simulink model "Furuta_Control_all_states_24_12_4am0x2810x29"  (R2023b)
settings: Solver=FixedStepAuto  StartTime=0.0  StopTime=inf  FixedStep=Ts  RelTol=1e-3
PreLoadFcn:
  | %myBusDef
StartFcn:
  | % Full path to the block
  | %blk = 'Furuta_Control/Bus Creator';
  | 
  | % Attach the event listener
  | %h = add_exec_event_listener(blk, ...
  | %         'PostOutputs', @displayBusdata);
values from neighbouring files (symbols this model uses):
  a = exp(-wc*Ts)    [Furuta_Constants.m]
  K2 = place(Ap2,Bp2,[-5 -4 -2+2j -2-2j])    [Furuta_Constants.m]
libraries: arduinolib x3, eeGeneralControl x2, arduinosensorlib x2
settings Model: ExtModeTrigDuration=2  Creator=Marcelo  LastModifiedBy=Omar Elshawaf
settings SolverCC: ZeroCrossControl=DisableAll  AlgebraicLoopSolver=TrustRegion
settings DataIOCC: ReturnWorkspaceOutputs=off
settings OptimizationCC: EnhancedBackFolding=on  PassReuseOutputArgsAs=Individual arguments  ZeroExternalMemoryAtStartup=off  ZeroInternalMemoryAtStartup=off  MaxStackSize=64  OptimizeBlockOrder=speed  DifferentSizesBufferReuse=on  OptimizationCustomize=off  EfficientTunableParamExpr=on
settings DebuggingCC: ParameterOverflowMsg=warning  ParameterTunabilityLossMsg=error  UnconnectedInputMsg=warning  UnconnectedOutputMsg=warning  UnconnectedLineMsg=warning  BusObjectLabelMismatch=error  ArithmeticOperatorsInVariantConditions=warning
settings HardwareCC: ProdBitPerPointer=32  ProdBitPerSizeT=32  ProdBitPerPtrDiffT=32  ProdLargestAtomicInteger=Long  ProdLargestAtomicFloat=Double  ProdWordSize=32  ProdHWDeviceType=ARM Compatible->ARM Cortex
settings ModelReferenceCC: EnableRefExpFcnMdlSchedulingChecks=on  ModelReferenceMinAlgLoopOccurrences=on
settings SFSimCC: SimUseLocalCustomCode=off  MATLABDynamicMemAlloc=off  CustomCodeUndefinedFunction=UseInterfaceOnly
settings RTWCC: Description=Embedded Coder  SystemTargetFile=ert.tlc  HardwareBoard=ESP32-WROOM(Arduino Compatible)  TLCOptions="-aInlineSetEventsForThisBaseRateFcn=TLC_FALSE -aSuppressMultiTaskScheduler=TLC_FALSE  -aRateBasedStepFcn=0"  TemplateMakefile=ert_default_tmf  RTWUseLocalCustomCode=off  Toolchain=ESP32
settings CodeAppCC: ForceParamTrailComments=on  IgnoreCustomStorageClasses=off  OperatorAnnotations=on  SimulinkDataObjDesc=on  SFDataObjDesc=on  InsertBlockDesc=on
settings ERTTargetCC: SupportContinuousTime=on  SupportVariableSizeSignals=on  ExtModeTransport=3  ExtModeStaticAlloc=on  ExtModeAutomaticAllocSize=off  ExtModeStaticAllocSize=65536  ExtModeMexFile=ext_xcp  ExtModeMexArgs=0 12 115200  ExtModeIntrfLevel=Level2 - Open

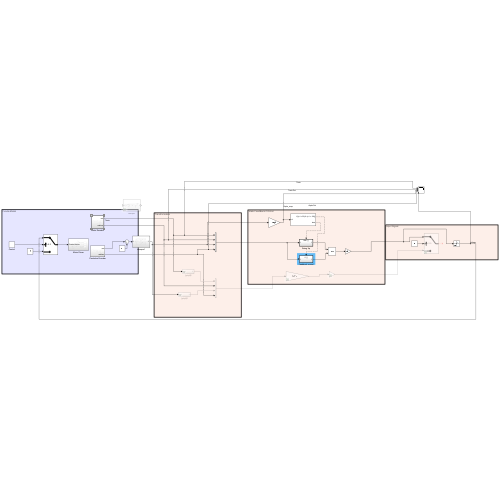
[thumbnail: Simulink's stored preview of the top-level diagram]
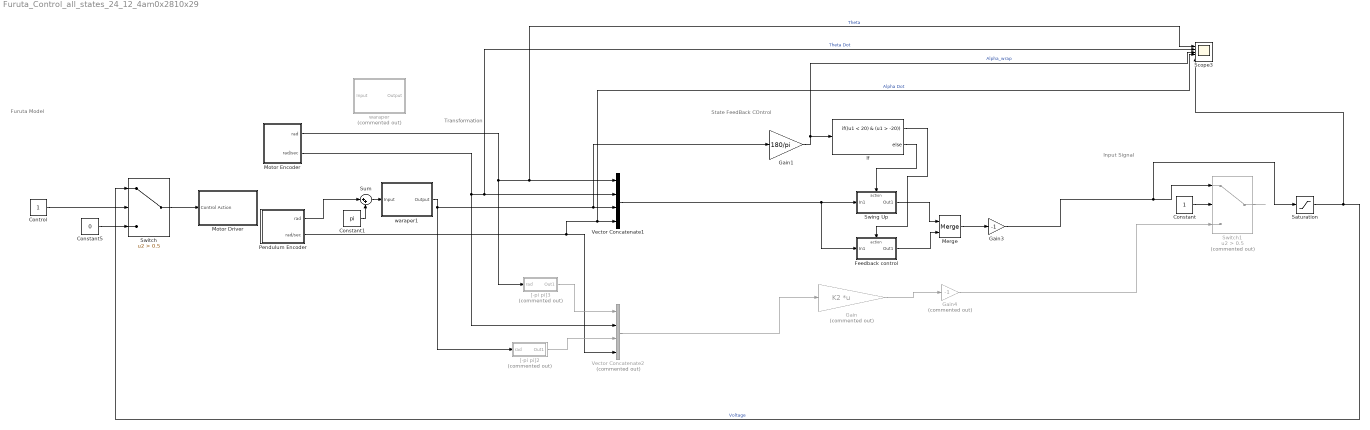
== system Furuta_Control_all_states_24_12_4am0x2810x29 ==
  note: State FeedBack COntrol
  note: Input Signal
  note: Furuta Model
  note: Transformation
  Constant : Constant  SampleTime=-1
  Constant1 : Constant  Value=pi  SampleTime=-1
  Constant5 : Constant  Value=0
  Control : Constant  SampleTime=-1
  Feedback control : Subsystem  TreatAsAtomicUnit=on
  Gain : Gain  Commented=on  Gain=K2  Multiplication=Matrix(K*u)
  Gain1 : Gain  Gain=180/pi
  Gain3 : Gain  Gain=-1
  Gain4 : Gain  Commented=on  Gain=-1
  If : If  IfExpression=(u1 < 20) & (u1 > -20)
  Merge : Merge
  Motor Driver : Subsystem
  Motor Encoder : Subsystem
  Pendulum Encoder : Subsystem
  Saturation : Saturate  UpperLimit=255  LowerLimit=-255
  Scope3 : Scope  NumInputPorts=5
  Sum : Sum  Inputs=|++
  Swing Up : Subsystem  TreatAsAtomicUnit=on
  Switch : Switch  Criteria=u2 > Threshold  Threshold=0.5  SaturateOnIntegerOverflow=off  InputSameDT=off
  Switch1 : Switch  Commented=on  Criteria=u2 > Threshold  Threshold=0.5  SaturateOnIntegerOverflow=off  InputSameDT=off
  Vector Concatenate1 : Concatenate  NumInputs=4  Mode=Multidimensional array
  Vector Concatenate2 : Concatenate  Commented=on  NumInputs=4  Mode=Multidimensional array
  "[-pi pi]2" : Subsystem  Commented=on
  "[-pi pi]3" : Subsystem  Commented=on
  waraper : Subsystem  Commented=on
  waraper1 : Subsystem
  wires:
  Swing Up/1(Out1) -> Merge/1
  Pendulum Encoder/2(rad/sec) -> Vector Concatenate2/4, Scope3/4, Vector Concatenate1/4  "Alpha Dot"
  Feedback control/1(Out1) -> Merge/2
  Control/1 -> Switch/2
  Constant5/1 -> Switch/3
  Sum/1 -> waraper1/1(Input)
  Vector Concatenate1/1 -> Feedback control/1(In1), Swing Up/1(In1)
  Gain1/1 -> Scope3/3, If/1  "Alpha_wrap"
  "[-pi pi]2"/1(Out1) -> Vector Concatenate2/3
  Motor Encoder/2(rad/sec) -> Vector Concatenate2/2, Vector Concatenate1/2, Scope3/2  "Theta Dot"
  Vector Concatenate2/1 -> Gain/1
  Saturation/1 -> Switch/1, Scope3/5  "Voltage"
  Switch1/1 -> ?
  Gain3/1 -> Saturation/1, Switch1/1
  Gain4/1 -> Switch1/3
  Merge/1 -> Gain3/1
  Constant/1 -> Switch1/2
  Switch/1 -> Motor Driver/1(Control Action)
  Gain/1 -> Gain4/1
  "[-pi pi]3"/1(Out1) -> Vector Concatenate2/1
  If/2 -> Swing Up/Action
  If/1 -> Feedback control/Action
  Constant1/1 -> Sum/2
  Pendulum Encoder/1(rad) -> Sum/1
  waraper1/1(Output) -> "[-pi pi]2"/1(rad), Gain1/1, Vector Concatenate1/3
  Motor Encoder/1(rad) -> Vector Concatenate1/1, Scope3/1, "[-pi pi]3"/1(rad)  "Theta"

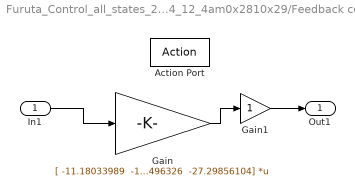
== system Furuta_Control_all_states_24_12_4am0x2810x29/Feedback control ==
  In1 : Inport
  Action Port : ActionPort  ActionPortLabel=if((u1 < 20) & (u1 > -20))
  Gain : Gain  Gain="[ -11.18033989  -17.56383192 -336.55496326  -27.29856104]"  Multiplication=Matrix(K*u)  ParamDataTypeStr=double  OutDataTypeStr=double
  Gain1 : Gain
  Out1 : Outport  VectorParamsAs1DForOutWhenUnconnected=off
  wires:
  In1/1 -> Gain/1
  Gain/1 -> Gain1/1
  Gain1/1 -> Out1/1

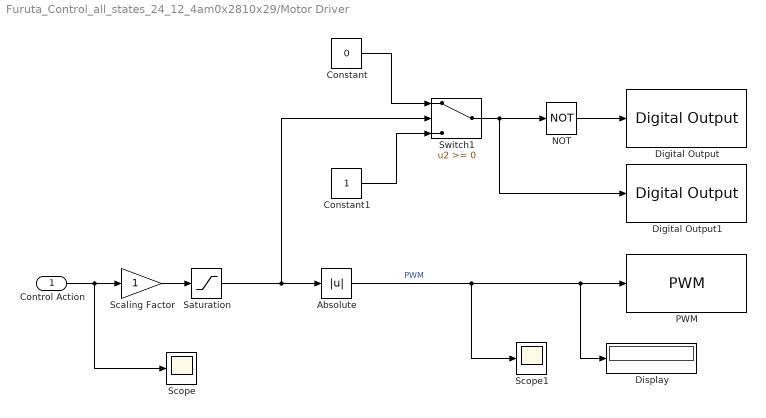
== system Furuta_Control_all_states_24_12_4am0x2810x29/Motor Driver ==
  Control Action : Inport
  Absolute : Abs  SaturateOnIntegerOverflow=off
  Constant : Constant  Value=0
  Constant1 : Constant
  Digital Output : arduinolib/Digital Output  pinNumber=26  Direction=output  blockPlatform=arduino
  Digital Output1 : arduinolib/Digital Output  pinNumber=19  Direction=output  blockPlatform=arduino
  Display : Display
  NOT : Logic  Operator=NOT  IconShape=distinctive  AllPortsSameDT=off  OutDataTypeStr=boolean
  PWM : arduinolib/PWM  pinNumber=12  frequencyType=Default  desiredFrequency=490.2  achievableFrequency=490.2
  Saturation : Saturate  UpperLimit=255  LowerLimit=-255
  Scaling Factor : Gain
  Scope : Scope
  Scope1 : Scope
  Switch1 : Switch  SaturateOnIntegerOverflow=off  InputSameDT=off
  wires:
  NOT/1 -> Digital Output/1
  Control Action/1 -> Scaling Factor/1, Scope/1
  Switch1/1 -> Digital Output1/1, NOT/1
  Constant/1 -> Switch1/1
  Constant1/1 -> Switch1/3
  Saturation/1 -> Switch1/2, Absolute/1
  Scaling Factor/1 -> Saturation/1
  Absolute/1 -> Scope1/1, Display/1, PWM/1  "PWM"

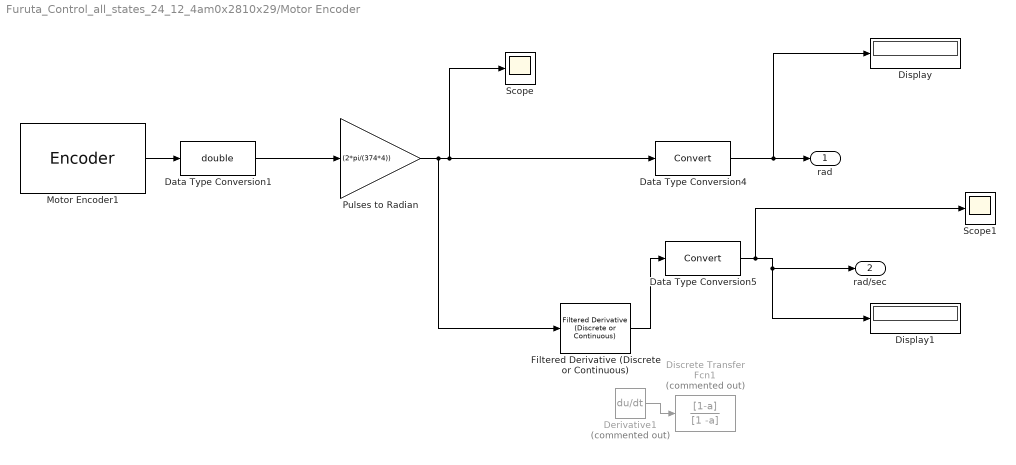
== system Furuta_Control_all_states_24_12_4am0x2810x29/Motor Encoder ==
  Data Type Conversion1 : DataTypeConversion  OutDataTypeStr=double  SaturateOnIntegerOverflow=off  RndMeth=Floor
  Data Type Conversion4 : DataTypeConversion  SaturateOnIntegerOverflow=off  RndMeth=Floor
  Data Type Conversion5 : DataTypeConversion  SaturateOnIntegerOverflow=off  RndMeth=Floor
  Derivative1 : Derivative  Commented=on
  Discrete Transfer Fcn1 : DiscreteTransferFcn  Commented=on  Numerator=[1-a]  Denominator=[1 -a]
  Display : Display
  Display1 : Display
  Filtered Derivative (Discrete or Continuous) : eeGeneralControl/Filtered Derivative (Discrete or Continuous)  K=1  T=0.01  B=inf  A=-inf  minRatio=10  init_option=Inherited from block input  x0=0  Ts=-1
  Motor Encoder1 : arduinosensorlib/Encoder  InputA=32  InputB=33  Mode=No reset  SampleTime=-1
  Pulses to Radian : Gain  Gain=(2*pi/(374*4))
  Scope : Scope
  Scope1 : Scope
  rad : Outport
  rad/sec : Outport  Port=2
  wires:
  Data Type Conversion1/1 -> Pulses to Radian/1
  Motor Encoder1/1 -> Data Type Conversion1/1
  Data Type Conversion4/1 -> Display/1, rad/1
  Data Type Conversion5/1 -> Scope1/1, rad/sec/1, Display1/1
  Filtered Derivative (Discrete or Continuous)/1 -> Data Type Conversion5/1
  Pulses to Radian/1 -> Filtered Derivative (Discrete or Continuous)/1, Data Type Conversion4/1, Scope/1
  Derivative1/1 -> Discrete Transfer Fcn1/1

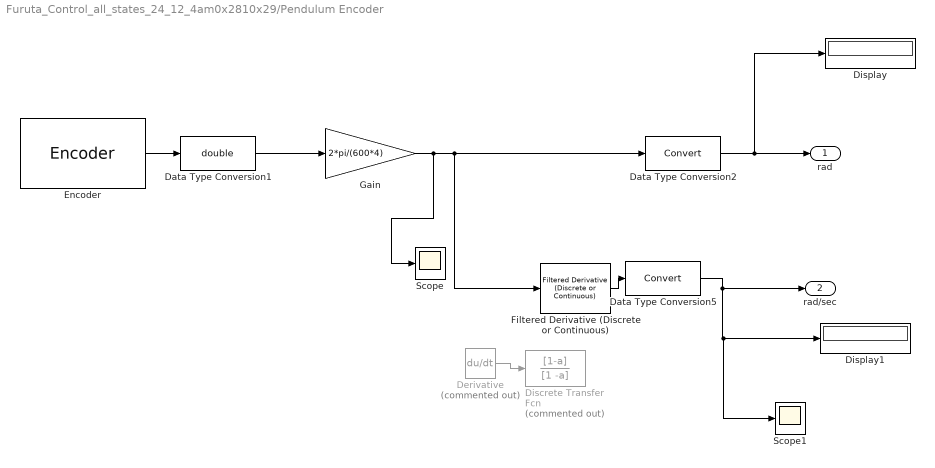
== system Furuta_Control_all_states_24_12_4am0x2810x29/Pendulum Encoder ==
  Data Type Conversion1 : DataTypeConversion  OutDataTypeStr=double  SaturateOnIntegerOverflow=off  RndMeth=Floor
  Data Type Conversion2 : DataTypeConversion  SaturateOnIntegerOverflow=off  RndMeth=Floor
  Data Type Conversion5 : DataTypeConversion  SaturateOnIntegerOverflow=off  RndMeth=Floor
  Derivative : Derivative  Commented=on
  Discrete Transfer Fcn : DiscreteTransferFcn  Commented=on  Numerator=[1-a]  Denominator=[1 -a]
  Display : Display
  Display1 : Display
  Encoder : arduinosensorlib/Encoder  InputA=25  InputB=27  Mode=No reset  SampleTime=-1
  Filtered Derivative (Discrete or Continuous) : eeGeneralControl/Filtered Derivative (Discrete or Continuous)  K=1  T=0.01  B=inf  A=-inf  minRatio=10  init_option=Inherited from block input  x0=0  Ts=-1
  Gain : Gain  Gain=2*pi/(600*4)
  Scope : Scope
  Scope1 : Scope
  rad : Outport
  rad/sec : Outport  Port=2
  wires:
  Data Type Conversion1/1 -> Gain/1
  Encoder/1 -> Data Type Conversion1/1
  Data Type Conversion2/1 -> Display/1, rad/1
  Data Type Conversion5/1 -> rad/sec/1, Scope1/1, Display1/1
  Filtered Derivative (Discrete or Continuous)/1 -> Data Type Conversion5/1
  Gain/1 -> Scope/1, Filtered Derivative (Discrete or Continuous)/1, Data Type Conversion2/1
  Derivative/1 -> Discrete Transfer Fcn/1

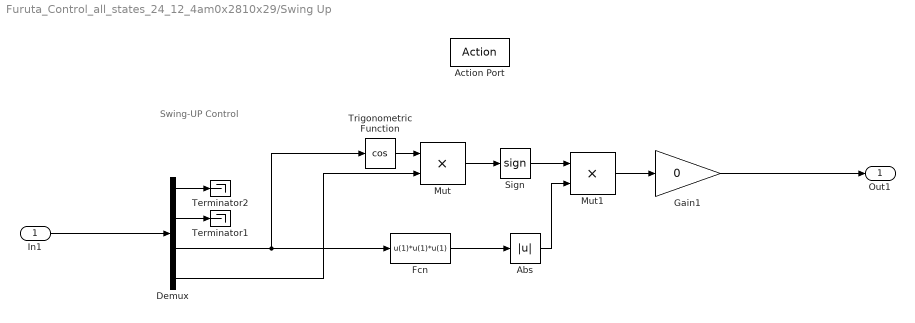
== system Furuta_Control_all_states_24_12_4am0x2810x29/Swing Up ==
  note: Swing-UP Control
  In1 : Inport
  Action Port : ActionPort  ActionPortLabel=else
  Abs : Abs  SaturateOnIntegerOverflow=off
  Demux : Demux
  Fcn : Fcn  Expr=u(1)*u(1)*u(1)
  Gain1 : Gain  Gain=0
  Mut : Product  Inputs=**
  Mut1 : Product  Inputs=**
  Sign : Signum
  Terminator1 : Terminator
  Terminator2 : Terminator
  Trigonometric Function : Trigonometry  Operator=cos
  Out1 : Outport  InitialOutput=0  VectorParamsAs1DForOutWhenUnconnected=off
  wires:
  Gain1/1 -> Out1/1
  Demux/2 -> Terminator1/1
  Demux/1 -> Terminator2/1
  Mut1/1 -> Gain1/1
  Fcn/1 -> Abs/1
  Trigonometric Function/1 -> Mut/1
  Demux/4 -> Mut/2
  Abs/1 -> Mut1/2
  Sign/1 -> Mut1/1
  Mut/1 -> Sign/1
  Demux/3 -> Fcn/1, Trigonometric Function/1
  In1/1 -> Demux/1

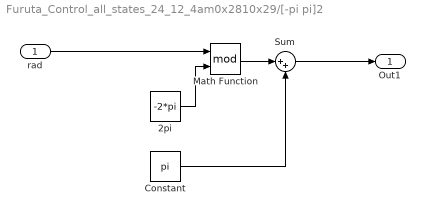
== system Furuta_Control_all_states_24_12_4am0x2810x29/[-pi pi]2 ==
  rad : Inport
  2pi : Constant  Value=-2*pi
  Constant : Constant  Value=pi
  Math Function : Math  Operator=mod  SignedPower=on
  Sum : Sum  Inputs=|++
  Out1 : Outport  VectorParamsAs1DForOutWhenUnconnected=off
  wires:
  2pi/1 -> Math Function/2
  rad/1 -> Math Function/1
  Math Function/1 -> Sum/1
  Constant/1 -> Sum/2
  Sum/1 -> Out1/1

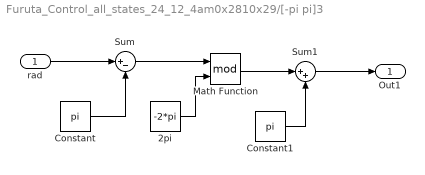
== system Furuta_Control_all_states_24_12_4am0x2810x29/[-pi pi]3 ==
  rad : Inport
  2pi : Constant  Value=-2*pi
  Constant : Constant  Value=pi
  Constant1 : Constant  Value=pi
  Math Function : Math  Operator=mod  SignedPower=on
  Sum : Sum  Inputs=|+-
  Sum1 : Sum  Inputs=|++
  Out1 : Outport  VectorParamsAs1DForOutWhenUnconnected=off
  wires:
  2pi/1 -> Math Function/2
  rad/1 -> Sum/1
  Sum/1 -> Math Function/1
  Constant/1 -> Sum/2
  Constant1/1 -> Sum1/2
  Sum1/1 -> Out1/1
  Math Function/1 -> Sum1/1

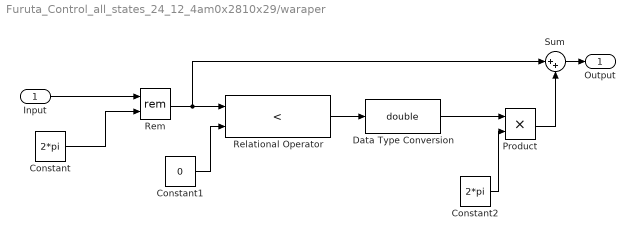
== system Furuta_Control_all_states_24_12_4am0x2810x29/waraper ==
  Input : Inport
  Constant : Constant  Value=2*pi
  Constant1 : Constant  Value=0
  Constant2 : Constant  Value=2*pi
  Data Type Conversion : DataTypeConversion  OutDataTypeStr=double  SaturateOnIntegerOverflow=off  RndMeth=Floor
  Product : Product
  Relational Operator : RelationalOperator  Operator=<  OutDataTypeStr=boolean  RndMeth=Simplest  InputSameDT=off
  Rem : Math  Operator=rem
  Sum : Sum  Inputs=|++
  Output : Outport
  wires:
  Constant/1 -> Rem/2
  Input/1 -> Rem/1
  Rem/1 -> Sum/1, Relational Operator/1
  Constant1/1 -> Relational Operator/2
  Product/1 -> Sum/2
  Relational Operator/1 -> Data Type Conversion/1
  Constant2/1 -> Product/2
  Sum/1 -> Output/1
  Data Type Conversion/1 -> Product/1

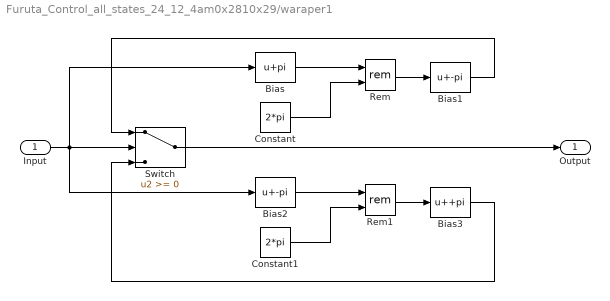
== system Furuta_Control_all_states_24_12_4am0x2810x29/waraper1 ==
  Input : Inport
  Bias : Bias  Bias=pi  SaturateOnIntegerOverflow=off
  Bias1 : Bias  Bias=-pi  SaturateOnIntegerOverflow=off
  Bias2 : Bias  Bias=-pi  SaturateOnIntegerOverflow=off
  Bias3 : Bias  Bias=+pi  SaturateOnIntegerOverflow=off
  Constant : Constant  Value=2*pi
  Constant1 : Constant  Value=2*pi
  Rem : Math  Operator=rem
  Rem1 : Math  Operator=rem
  Switch : Switch  SaturateOnIntegerOverflow=off  InputSameDT=off
  Output : Outport
  wires:
  Constant/1 -> Rem/2
  Bias/1 -> Rem/1
  Input/1 -> Bias/1, Bias2/1, Switch/2
  Bias3/1 -> Switch/3
  Bias2/1 -> Rem1/1
  Rem1/1 -> Bias3/1
  Constant1/1 -> Rem1/2
  Switch/1 -> Output/1
  Rem/1 -> Bias1/1
  Bias1/1 -> Switch/1
